simulink model "base_evaluation_1008_24b"  (R2016b)
settings: Solver=FixedStepAuto  StartTime=0.0  StopTime=10.0  RelTol=1e-3
settings Model: Creator=Cheng  LastModifiedBy=kensh
settings DataIOCC: ReturnWorkspaceOutputs=on
settings OptimizationCC: DefaultParameterBehavior=Inlined
settings DebuggingCC: ParameterTunabilityLossMsg=error  UnconnectedInputMsg=none  UnconnectedOutputMsg=none  UnconnectedLineMsg=none
settings ModelReferenceCC: EnableRefExpFcnMdlSchedulingChecks=off
settings SFSimCC: SimUseLocalCustomCode=on
settings RTWCC: SystemTargetFile=ert.tlc  TemplateMakefile=ert_default_tmf  Description=Embedded Coder  GenerateReport=on  RTWUseLocalCustomCode=on  IncludeHyperlinkInReport=on  LaunchReport=on  GenerateTraceInfo=on  GenerateTraceReport=on  GenerateTraceReportSl=on  GenerateTraceReportSf=on  GenerateTraceReportEml=on
settings CodeAppCC: ForceParamTrailComments=on  IgnoreCustomStorageClasses=off  OperatorAnnotations=on  SimulinkDataObjDesc=on  SFDataObjDesc=on  MATLABFcnDesc=on  InsertBlockDesc=on  MATLABSourceComments=on
settings ERTTargetCC: TargetLangStandard=C99 (ISO)  GenerateSampleERTMain=on  InlinedParameterPlacement=NonHierarchical  ERTCustomFileTemplate=example_file_process.tlc

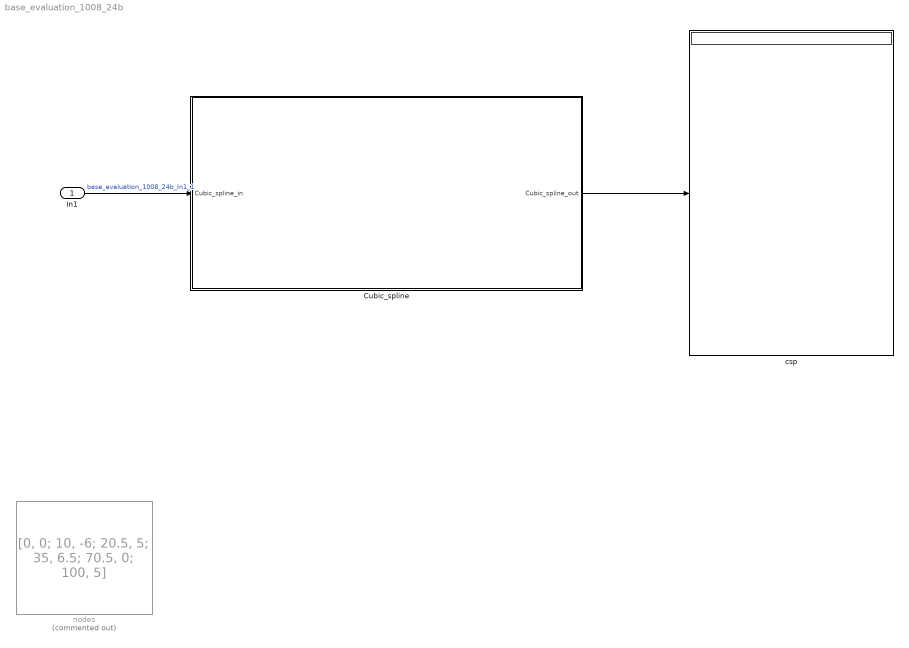
== system base_evaluation_1008_24b ==
  In1 : Inport
  Cubic_spline : Subsystem
  csp : Display
  nodes : Constant  Commented=on  Value=[0, 0; 10, -6; 20.5, 5; 35, 6.5; 70.5, 0; 100, 5]
  wires:
  Cubic_spline/1(Cubic_spline_out) -> csp/1
  In1/1 -> Cubic_spline/1(Cubic_spline_in)  "base_evaluation_1008_24b_In1_1"

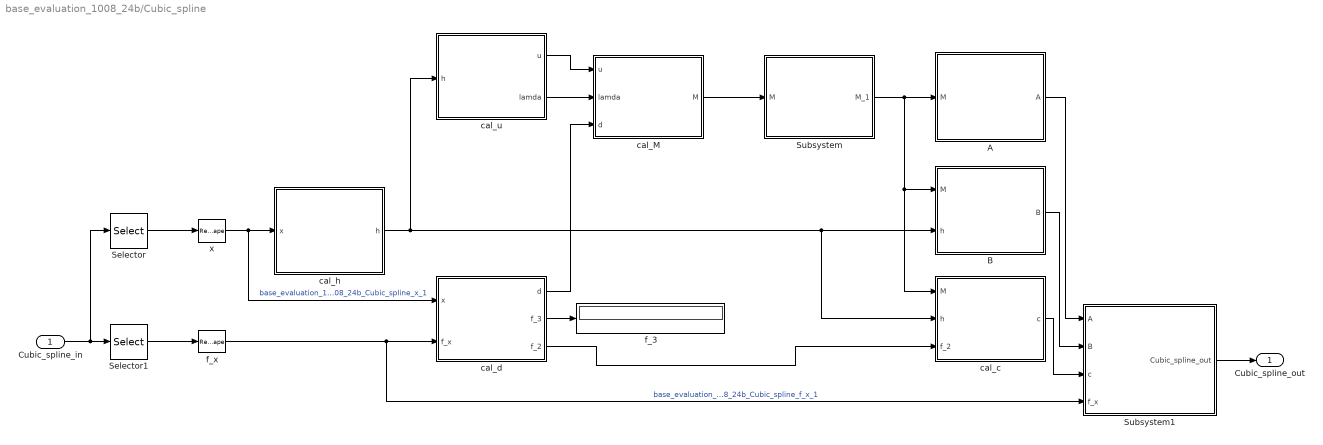
== system base_evaluation_1008_24b/Cubic_spline ==
  Cubic_spline_in : Inport
  A : Subsystem
  B : Subsystem
  Selector : Selector  NumberOfDimensions=2  InputPortWidth=3  IndexOptions=Select all,Index vector (dialog)  Indices=1,1  OutputSizes=1,1
  Selector1 : Selector  NumberOfDimensions=2  InputPortWidth=3  IndexOptions=Select all,Index vector (dialog)  Indices=1,2  OutputSizes=1,1
  Subsystem : Subsystem
  Subsystem1 : Subsystem
  cal_M : Subsystem
  cal_c : Subsystem
  cal_d : Subsystem
  cal_h : Subsystem
  cal_u : Subsystem
  f_3 : Display
  f_x : Reshape  OutputDimensionality=Row vector (2-D)
  x : Reshape  OutputDimensionality=Row vector (2-D)
  Cubic_spline_out : Outport
  wires:
  Cubic_spline_in/1 -> Selector1/1, Selector/1
  f_x/1 -> Subsystem1/4(f_x), cal_d/2(f_x)  "base_evaluation_1008_24b_Cubic_spline_f_x_1"
  Selector1/1 -> f_x/1
  Selector/1 -> x/1
  x/1 -> cal_d/1(x), cal_h/1(x)  "base_evaluation_1008_24b_Cubic_spline_x_1"
  cal_M/1(M) -> Subsystem/1(M)
  cal_h/1(h) -> cal_c/2(h), B/2(h), cal_u/1(h)
  cal_u/1(u) -> cal_M/1(u)
  cal_c/1(c) -> Subsystem1/3(c)
  cal_u/2(lamda) -> cal_M/2(lamda)
  cal_d/1(d) -> cal_M/3(d)
  cal_d/2(f_3) -> f_3/1
  cal_d/3(f_2) -> cal_c/3(f_2)
  Subsystem/1(M_1) -> B/1(M), cal_c/1(M), A/1(M)
  A/1(A) -> Subsystem1/1(A)
  B/1(B) -> Subsystem1/2(B)
  Subsystem1/1(Cubic_spline_out) -> Cubic_spline_out/1

== system base_evaluation_1008_24b/Cubic_spline/A ==
  M : Inport
  Gain{,1..4} (5 alike) : Gain  Gain=0.5
  M1 : Selector  InputPortWidth=6  IndexOptions=Index vector (dialog)  Indices=[1]  OutputSizes=1
  M2 : Selector  InputPortWidth=6  IndexOptions=Index vector (dialog)  Indices=[2]  OutputSizes=1
  M3 : Selector  InputPortWidth=6  IndexOptions=Index vector (dialog)  Indices=[3]  OutputSizes=1
  M4 : Selector  InputPortWidth=6  IndexOptions=Index vector (dialog)  Indices=[4]  OutputSizes=1
  M5 : Selector  InputPortWidth=6  IndexOptions=Index vector (dialog)  Indices=[5]  OutputSizes=1
  Mux : Mux  Inputs=5
  Reshape : Reshape  OutputDimensionality=Row vector (2-D)
  A : Outport
  wires:
  M3/1 -> Gain2/1
  M4/1 -> Gain3/1
  M/1 -> M5/1, M4/1, M3/1, M2/1, M1/1
  M2/1 -> Gain1/1
  M1/1 -> Gain/1
  M5/1 -> Gain4/1
  Gain/1 -> Mux/1  "base_evaluation_1008_24b_Cubic_spline_A_Gain_1"
  Gain1/1 -> Mux/2  "base_evaluation_1008_24b_Cubic_spline_A_Gain1_1"
  Gain2/1 -> Mux/3  "base_evaluation_1008_24b_Cubic_spline_A_Gain2_1"
  Gain3/1 -> Mux/4  "base_evaluation_1008_24b_Cubic_spline_A_Gain3_1"
  Gain4/1 -> Mux/5  "base_evaluation_1008_24b_Cubic_spline_A_Gain4_1"
  Mux/1 -> Reshape/1
  Reshape/1 -> A/1  "base_evaluation_1008_24b_Cubic_spline_A_Reshape_1"

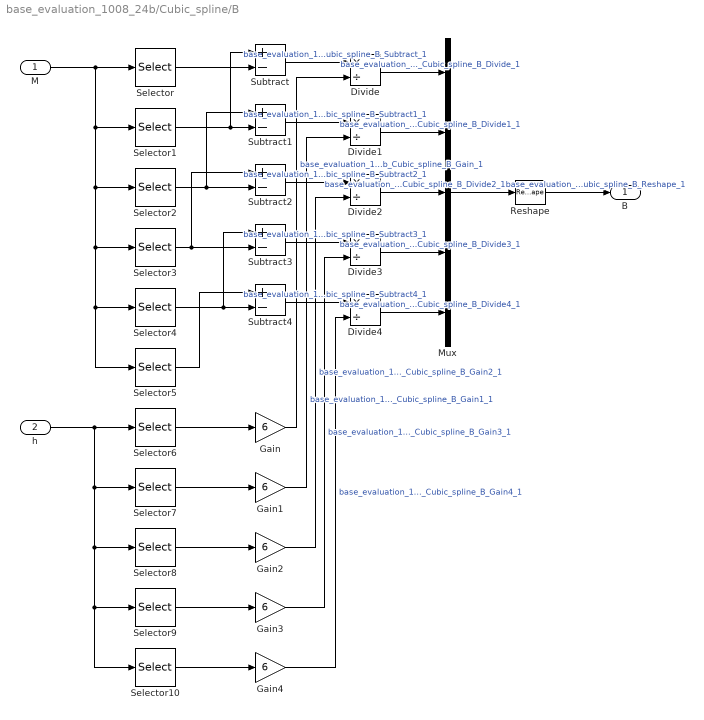
== system base_evaluation_1008_24b/Cubic_spline/B ==
  M : Inport
  h : Inport  Port=2
  Divide{,1..4} (5 alike) : Product  Inputs=*/
  Gain{,1..4} (5 alike) : Gain  Gain=6
  Mux : Mux  Inputs=5
  Reshape : Reshape  OutputDimensionality=Row vector (2-D)
  Selector : Selector  InputPortWidth=6  IndexOptions=Index vector (dialog)  Indices=[1]  OutputSizes=1
  Selector1 : Selector  InputPortWidth=6  IndexOptions=Index vector (dialog)  Indices=[2]  OutputSizes=1
  Selector10 : Selector  InputPortWidth=5  IndexOptions=Index vector (dialog)  Indices=[5]  OutputSizes=1
  Selector2 : Selector  InputPortWidth=6  IndexOptions=Index vector (dialog)  Indices=[3]  OutputSizes=1
  Selector3 : Selector  InputPortWidth=6  IndexOptions=Index vector (dialog)  Indices=[4]  OutputSizes=1
  Selector4 : Selector  InputPortWidth=6  IndexOptions=Index vector (dialog)  Indices=[5]  OutputSizes=1
  Selector5 : Selector  InputPortWidth=6  IndexOptions=Index vector (dialog)  Indices=[6]  OutputSizes=1
  Selector6 : Selector  InputPortWidth=5  IndexOptions=Index vector (dialog)  Indices=[1]  OutputSizes=1
  Selector7 : Selector  InputPortWidth=5  IndexOptions=Index vector (dialog)  Indices=[2]  OutputSizes=1
  Selector8 : Selector  InputPortWidth=5  IndexOptions=Index vector (dialog)  Indices=[3]  OutputSizes=1
  Selector9 : Selector  InputPortWidth=5  IndexOptions=Index vector (dialog)  Indices=[4]  OutputSizes=1
  Subtract{,1..4} (5 alike) : Sum  Inputs=+-
  B : Outport
  wires:
  h/1 -> Selector10/1, Selector9/1, Selector8/1, Selector7/1, Selector6/1
  M/1 -> Selector5/1, Selector4/1, Selector3/1, Selector2/1, Selector1/1, Selector/1
  Selector1/1 -> Subtract1/2, Subtract/1
  Selector/1 -> Subtract/2
  Selector2/1 -> Subtract2/2, Subtract1/1
  Selector3/1 -> Subtract3/2, Subtract2/1
  Selector6/1 -> Gain/1
  Selector7/1 -> Gain1/1
  Selector8/1 -> Gain2/1
  Subtract/1 -> Divide/1  "base_evaluation_1008_24b_Cubic_spline_B_Subtract_1"
  Gain/1 -> Divide/2  "base_evaluation_1008_24b_Cubic_spline_B_Gain_1"
  Subtract1/1 -> Divide1/1  "base_evaluation_1008_24b_Cubic_spline_B_Subtract1_1"
  Gain1/1 -> Divide1/2  "base_evaluation_1008_24b_Cubic_spline_B_Gain1_1"
  Subtract2/1 -> Divide2/1  "base_evaluation_1008_24b_Cubic_spline_B_Subtract2_1"
  Gain2/1 -> Divide2/2  "base_evaluation_1008_24b_Cubic_spline_B_Gain2_1"
  Divide/1 -> Mux/1  "base_evaluation_1008_24b_Cubic_spline_B_Divide_1"
  Divide1/1 -> Mux/2  "base_evaluation_1008_24b_Cubic_spline_B_Divide1_1"
  Divide2/1 -> Mux/3  "base_evaluation_1008_24b_Cubic_spline_B_Divide2_1"
  Mux/1 -> Reshape/1
  Reshape/1 -> B/1  "base_evaluation_1008_24b_Cubic_spline_B_Reshape_1"
  Selector4/1 -> Subtract4/2, Subtract3/1
  Selector5/1 -> Subtract4/1
  Selector9/1 -> Gain3/1
  Selector10/1 -> Gain4/1
  Divide3/1 -> Mux/4  "base_evaluation_1008_24b_Cubic_spline_B_Divide3_1"
  Divide4/1 -> Mux/5  "base_evaluation_1008_24b_Cubic_spline_B_Divide4_1"
  Subtract3/1 -> Divide3/1  "base_evaluation_1008_24b_Cubic_spline_B_Subtract3_1"
  Subtract4/1 -> Divide4/1  "base_evaluation_1008_24b_Cubic_spline_B_Subtract4_1"
  Gain3/1 -> Divide3/2  "base_evaluation_1008_24b_Cubic_spline_B_Gain3_1"
  Gain4/1 -> Divide4/2  "base_evaluation_1008_24b_Cubic_spline_B_Gain4_1"

== system base_evaluation_1008_24b/Cubic_spline/Subsystem ==
  M : Inport
  Constant : Constant  Value=0
  Constant1 : Constant  Value=0
  M1 : Selector  InputPortWidth=4  IndexOptions=Index vector (dialog)  Indices=[1]  OutputSizes=1
  M2 : Selector  InputPortWidth=4  IndexOptions=Index vector (dialog)  Indices=[2]  OutputSizes=1
  M3 : Selector  InputPortWidth=4  IndexOptions=Index vector (dialog)  Indices=[3]  OutputSizes=1
  M4 : Selector  InputPortWidth=4  IndexOptions=Index vector (dialog)  Indices=[4]  OutputSizes=1
  Mux : Mux  Inputs=6
  Reshape : Reshape  OutputDimensionality=Column vector (2-D)
  M_1 : Outport
  wires:
  Mux/1 -> Reshape/1
  Constant/1 -> Mux/1  "base_evaluation_1008_24b_Cubic_spline_Subsystem_Constant_1"
  M1/1 -> Mux/2
  Constant1/1 -> Mux/6  "base_evaluation_1008_24b_Cubic_spline_Subsystem_Constant1_1"
  M2/1 -> Mux/3
  Reshape/1 -> M_1/1  "base_evaluation_1008_24b_Cubic_spline_Subsystem_Reshape_1"
  M3/1 -> Mux/4
  M4/1 -> Mux/5
  M/1 -> M4/1, M3/1, M2/1, M1/1

== system base_evaluation_1008_24b/Cubic_spline/Subsystem1 ==
  A : Inport
  B : Inport  Port=2
  c : Inport  Port=3
  f_x : Inport  Port=4
  MatrixConcatenate : Concatenate  NumInputs=5  Mode=Multidimensional array
  Subsystem : Subsystem
  Subsystem1 : Subsystem
  Subsystem2 : Subsystem
  Subsystem3 : Subsystem
  Subsystem4 : Subsystem
  Cubic_spline_out : Outport
  wires:
  A/1 -> Subsystem1/1(A), Subsystem2/1(A), Subsystem4/1(A), Subsystem3/1(A), Subsystem/1(A)
  B/1 -> Subsystem/2(B), Subsystem1/2(B), Subsystem2/2(B), Subsystem4/2(B), Subsystem3/2(B)
  c/1 -> Subsystem/3(c), Subsystem1/3(c), Subsystem2/3(c), Subsystem4/3(c), Subsystem3/3(c)
  f_x/1 -> Subsystem/4(f_x), Subsystem1/4(f_x), Subsystem2/4(f_x), Subsystem4/4(f_x), Subsystem3/4(f_x)
  Subsystem/1(1) -> MatrixConcatenate/1
  Subsystem1/1(2) -> MatrixConcatenate/2
  Subsystem2/1(3) -> MatrixConcatenate/3
  Subsystem3/1(4) -> MatrixConcatenate/4
  Subsystem4/1(5) -> MatrixConcatenate/5
  MatrixConcatenate/1 -> Cubic_spline_out/1  "base_evaluation_1008_24b_Cubic_spline_Subsystem1_MatrixConcatenate_1"

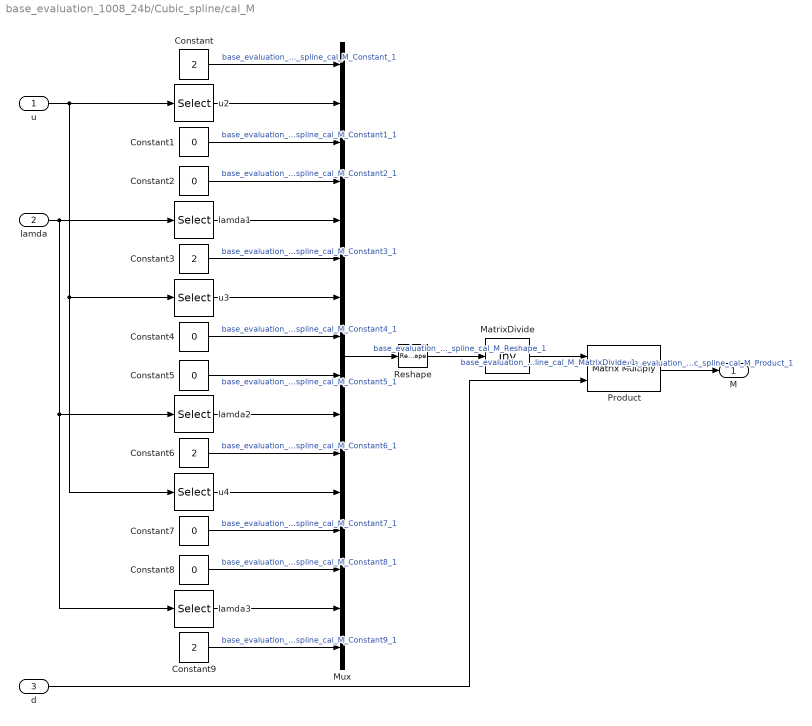
== system base_evaluation_1008_24b/Cubic_spline/cal_M ==
  u : Inport
  lamda : Inport  Port=2
  d : Inport  Port=3
  Constant{,3,6,9} (4 alike) : Constant  Value=2
  Constant{1..2,4..5,7..8} (6 alike) : Constant  Value=0
  MatrixDivide : Product  Inputs=/  Multiplication=Matrix(*)
  Mux : Mux  Inputs=16
  Product : Product  Multiplication=Matrix(*)
  Reshape : Reshape  OutputDimensionality=Customize  OutputDimensions=[4,4]
  lamda1 : Selector  InputPortWidth=4  IndexOptions=Index vector (dialog)  Indices=[1]  OutputSizes=1
  lamda2 : Selector  InputPortWidth=4  IndexOptions=Index vector (dialog)  Indices=[2]  OutputSizes=1
  lamda3 : Selector  InputPortWidth=4  IndexOptions=Index vector (dialog)  Indices=[3]  OutputSizes=1
  u2 : Selector  InputPortWidth=4  IndexOptions=Index vector (dialog)  Indices=[2]  OutputSizes=1
  u3 : Selector  InputPortWidth=4  IndexOptions=Index vector (dialog)  Indices=[3]  OutputSizes=1
  u4 : Selector  InputPortWidth=4  IndexOptions=Index vector (dialog)  Indices=[4]  OutputSizes=1
  M : Outport
  wires:
  u/1 -> u2/1, u4/1, u3/1
  Mux/1 -> Reshape/1
  Constant/1 -> Mux/1  "base_evaluation_1008_24b_Cubic_spline_cal_M_Constant_1"
  Product/1 -> M/1  "base_evaluation_1008_24b_Cubic_spline_cal_M_Product_1"
  Constant1/1 -> Mux/3  "base_evaluation_1008_24b_Cubic_spline_cal_M_Constant1_1"
  Constant2/1 -> Mux/4  "base_evaluation_1008_24b_Cubic_spline_cal_M_Constant2_1"
  u2/1 -> Mux/2
  lamda1/1 -> Mux/5
  Constant3/1 -> Mux/6  "base_evaluation_1008_24b_Cubic_spline_cal_M_Constant3_1"
  u3/1 -> Mux/7
  Constant4/1 -> Mux/8  "base_evaluation_1008_24b_Cubic_spline_cal_M_Constant4_1"
  Constant5/1 -> Mux/9  "base_evaluation_1008_24b_Cubic_spline_cal_M_Constant5_1"
  lamda/1 -> lamda3/1, lamda2/1, lamda1/1
  lamda2/1 -> Mux/10
  Constant6/1 -> Mux/11  "base_evaluation_1008_24b_Cubic_spline_cal_M_Constant6_1"
  u4/1 -> Mux/12
  Constant7/1 -> Mux/13  "base_evaluation_1008_24b_Cubic_spline_cal_M_Constant7_1"
  Constant8/1 -> Mux/14  "base_evaluation_1008_24b_Cubic_spline_cal_M_Constant8_1"
  lamda3/1 -> Mux/15
  Constant9/1 -> Mux/16  "base_evaluation_1008_24b_Cubic_spline_cal_M_Constant9_1"
  Reshape/1 -> MatrixDivide/1  "base_evaluation_1008_24b_Cubic_spline_cal_M_Reshape_1"
  d/1 -> Product/2
  MatrixDivide/1 -> Product/1  "base_evaluation_1008_24b_Cubic_spline_cal_M_MatrixDivide_1"

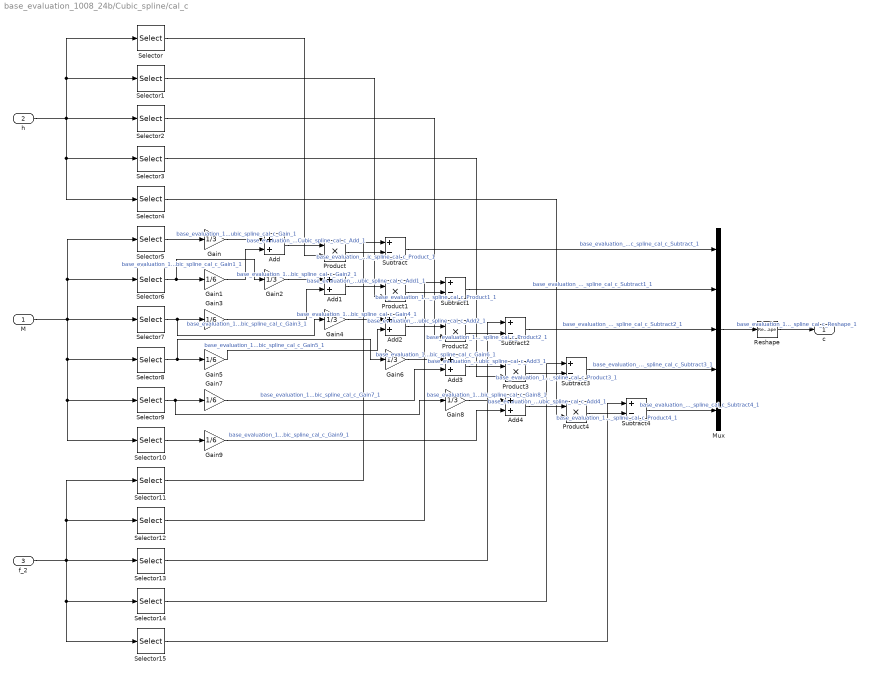
== system base_evaluation_1008_24b/Cubic_spline/cal_c ==
  M : Inport
  h : Inport  Port=2
  f_2 : Inport  Port=3
  Add{,1..4} (5 alike) : Sum
  Gain{,2,4,6,8} (5 alike) : Gain  Gain=1/3
  Gain{1,3,5,7,9} (5 alike) : Gain  Gain=1/6
  Mux : Mux  Inputs=5
  Product{,1..4} (5 alike) : Product
  Reshape : Reshape  OutputDimensionality=Row vector (2-D)
  Selector : Selector  InputPortWidth=5  IndexOptions=Index vector (dialog)  Indices=[1]  OutputSizes=1
  Selector1 : Selector  InputPortWidth=5  IndexOptions=Index vector (dialog)  Indices=[2]  OutputSizes=1
  Selector10 : Selector  InputPortWidth=6  IndexOptions=Index vector (dialog)  Indices=[6]  OutputSizes=1
  Selector11 : Selector  InputPortWidth=5  IndexOptions=Index vector (dialog)  Indices=[1]  OutputSizes=1
  Selector12 : Selector  InputPortWidth=5  IndexOptions=Index vector (dialog)  Indices=[2]  OutputSizes=1
  Selector13 : Selector  InputPortWidth=5  IndexOptions=Index vector (dialog)  Indices=[3]  OutputSizes=1
  Selector14 : Selector  InputPortWidth=5  IndexOptions=Index vector (dialog)  Indices=[4]  OutputSizes=1
  Selector15 : Selector  InputPortWidth=5  IndexOptions=Index vector (dialog)  Indices=[5]  OutputSizes=1
  Selector2 : Selector  InputPortWidth=5  IndexOptions=Index vector (dialog)  Indices=[3]  OutputSizes=1
  Selector3 : Selector  InputPortWidth=5  IndexOptions=Index vector (dialog)  Indices=[4]  OutputSizes=1
  Selector4 : Selector  InputPortWidth=5  IndexOptions=Index vector (dialog)  Indices=[5]  OutputSizes=1
  Selector5 : Selector  InputPortWidth=6  IndexOptions=Index vector (dialog)  Indices=[1]  OutputSizes=1
  Selector6 : Selector  InputPortWidth=6  IndexOptions=Index vector (dialog)  Indices=[2]  OutputSizes=1
  Selector7 : Selector  InputPortWidth=6  IndexOptions=Index vector (dialog)  Indices=[3]  OutputSizes=1
  Selector8 : Selector  InputPortWidth=6  IndexOptions=Index vector (dialog)  Indices=[4]  OutputSizes=1
  Selector9 : Selector  InputPortWidth=6  IndexOptions=Index vector (dialog)  Indices=[5]  OutputSizes=1
  Subtract{,1..4} (5 alike) : Sum  Inputs=+-
  c : Outport
  wires:
  Selector2/1 -> Product2/2
  Selector6/1 -> Gain2/1, Gain1/1
  Gain3/1 -> Add1/2  "base_evaluation_1008_24b_Cubic_spline_cal_c_Gain3_1"
  Gain/1 -> Add/1  "base_evaluation_1008_24b_Cubic_spline_cal_c_Gain_1"
  Selector7/1 -> Gain3/1, Gain4/1
  f_2/1 -> Selector11/1, Selector12/1, Selector15/1, Selector14/1, Selector13/1
  Add1/1 -> Product1/1  "base_evaluation_1008_24b_Cubic_spline_cal_c_Add1_1"
  Selector1/1 -> Product1/2
  M/1 -> Selector8/1, Selector9/1, Selector10/1, Selector7/1, Selector6/1, Selector5/1
  Subtract1/1 -> Mux/2  "base_evaluation_1008_24b_Cubic_spline_cal_c_Subtract1_1"
  Reshape/1 -> c/1  "base_evaluation_1008_24b_Cubic_spline_cal_c_Reshape_1"
  Gain1/1 -> Add/2  "base_evaluation_1008_24b_Cubic_spline_cal_c_Gain1_1"
  Add2/1 -> Product2/1  "base_evaluation_1008_24b_Cubic_spline_cal_c_Add2_1"
  Selector/1 -> Product/2
  Gain2/1 -> Add1/1  "base_evaluation_1008_24b_Cubic_spline_cal_c_Gain2_1"
  Selector5/1 -> Gain/1
  Subtract/1 -> Mux/1  "base_evaluation_1008_24b_Cubic_spline_cal_c_Subtract_1"
  Subtract2/1 -> Mux/3  "base_evaluation_1008_24b_Cubic_spline_cal_c_Subtract2_1"
  Selector13/1 -> Subtract2/1
  Gain4/1 -> Add2/1  "base_evaluation_1008_24b_Cubic_spline_cal_c_Gain4_1"
  Add/1 -> Product/1  "base_evaluation_1008_24b_Cubic_spline_cal_c_Add_1"
  Selector12/1 -> Subtract1/1
  h/1 -> Selector4/1, Selector3/1, Selector/1, Selector1/1, Selector2/1
  Selector11/1 -> Subtract/1
  Product2/1 -> Subtract2/2  "base_evaluation_1008_24b_Cubic_spline_cal_c_Product2_1"
  Product1/1 -> Subtract1/2  "base_evaluation_1008_24b_Cubic_spline_cal_c_Product1_1"
  Selector8/1 -> Gain6/1, Gain5/1
  Mux/1 -> Reshape/1
  Gain5/1 -> Add2/2  "base_evaluation_1008_24b_Cubic_spline_cal_c_Gain5_1"
  Product/1 -> Subtract/2  "base_evaluation_1008_24b_Cubic_spline_cal_c_Product_1"
  Selector9/1 -> Gain8/1, Gain7/1
  Gain6/1 -> Add3/1  "base_evaluation_1008_24b_Cubic_spline_cal_c_Gain6_1"
  Gain7/1 -> Add3/2  "base_evaluation_1008_24b_Cubic_spline_cal_c_Gain7_1"
  Add3/1 -> Product3/1  "base_evaluation_1008_24b_Cubic_spline_cal_c_Add3_1"
  Selector3/1 -> Product3/2
  Product3/1 -> Subtract3/2  "base_evaluation_1008_24b_Cubic_spline_cal_c_Product3_1"
  Selector14/1 -> Subtract3/1
  Selector10/1 -> Gain9/1
  Gain9/1 -> Add4/2  "base_evaluation_1008_24b_Cubic_spline_cal_c_Gain9_1"
  Gain8/1 -> Add4/1  "base_evaluation_1008_24b_Cubic_spline_cal_c_Gain8_1"
  Add4/1 -> Product4/1  "base_evaluation_1008_24b_Cubic_spline_cal_c_Add4_1"
  Selector4/1 -> Product4/2
  Product4/1 -> Subtract4/2  "base_evaluation_1008_24b_Cubic_spline_cal_c_Product4_1"
  Subtract3/1 -> Mux/4  "base_evaluation_1008_24b_Cubic_spline_cal_c_Subtract3_1"
  Selector15/1 -> Subtract4/1
  Subtract4/1 -> Mux/5  "base_evaluation_1008_24b_Cubic_spline_cal_c_Subtract4_1"

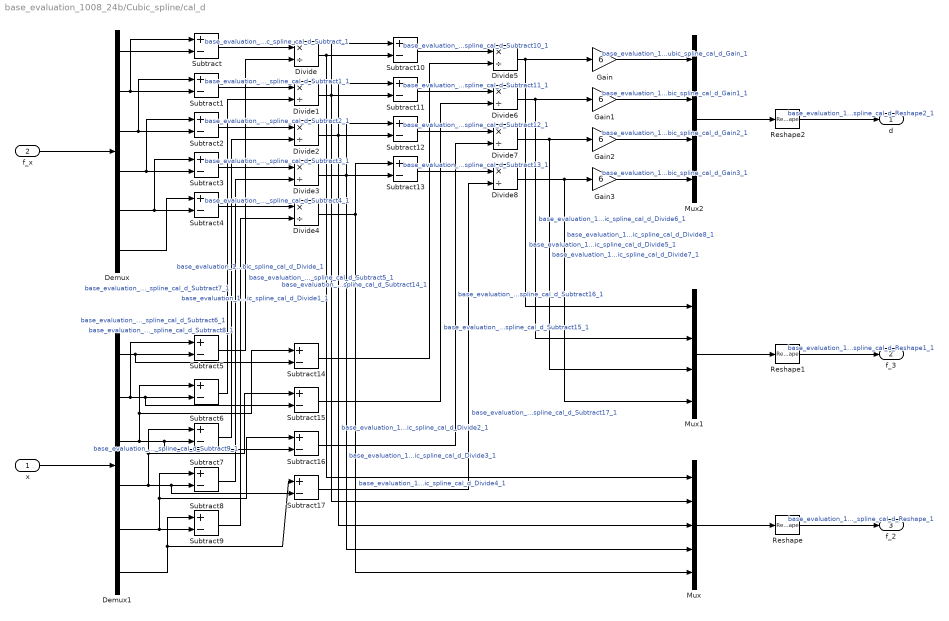
== system base_evaluation_1008_24b/Cubic_spline/cal_d ==
  x : Inport
  f_x : Inport  Port=2
  Demux : Demux  Outputs=6
  Demux1 : Demux  Outputs=6
  Divide{,1..8} (9 alike) : Product  Inputs=*/
  Gain{,1..3} (4 alike) : Gain  Gain=6
  Mux : Mux  Inputs=5
  Mux1 : Mux
  Mux2 : Mux
  Reshape : Reshape  OutputDimensionality=Row vector (2-D)
  Reshape1 : Reshape  OutputDimensionality=Row vector (2-D)
  Reshape2 : Reshape  OutputDimensionality=Column vector (2-D)
  Subtract{,1..17} (18 alike) : Sum  Inputs=+-
  d : Outport
  f_3 : Outport  Port=2
  f_2 : Outport  Port=3
  wires:
  f_x/1 -> Demux/1
  Demux1/2 -> Subtract6/2, Subtract15/2, Subtract5/1
  Demux/2 -> Subtract1/2, Subtract/1
  Mux/1 -> Reshape/1
  Subtract11/1 -> Divide6/1  "base_evaluation_1008_24b_Cubic_spline_cal_d_Subtract11_1"
  Subtract1/1 -> Divide1/1  "base_evaluation_1008_24b_Cubic_spline_cal_d_Subtract1_1"
  Demux/4 -> Subtract3/2, Subtract2/1
  Demux1/1 -> Subtract14/2, Subtract5/2
  Mux1/1 -> Reshape1/1
  Demux/3 -> Subtract2/2, Subtract1/1
  Divide2/1 -> Mux/3, Subtract12/2, Subtract11/1  "base_evaluation_1008_24b_Cubic_spline_cal_d_Divide2_1"
  Reshape1/1 -> f_3/1  "base_evaluation_1008_24b_Cubic_spline_cal_d_Reshape1_1"
  Divide1/1 -> Mux/2, Subtract11/2, Subtract10/1  "base_evaluation_1008_24b_Cubic_spline_cal_d_Divide1_1"
  Divide/1 -> Subtract10/2, Mux/1  "base_evaluation_1008_24b_Cubic_spline_cal_d_Divide_1"
  Divide6/1 -> Gain1/1, Mux1/2  "base_evaluation_1008_24b_Cubic_spline_cal_d_Divide6_1"
  Divide5/1 -> Gain/1, Mux1/1  "base_evaluation_1008_24b_Cubic_spline_cal_d_Divide5_1"
  Demux1/4 -> Subtract17/2, Subtract8/2, Subtract7/1, Subtract15/1
  Subtract6/1 -> Divide1/2  "base_evaluation_1008_24b_Cubic_spline_cal_d_Subtract6_1"
  Subtract10/1 -> Divide5/1  "base_evaluation_1008_24b_Cubic_spline_cal_d_Subtract10_1"
  Subtract2/1 -> Divide2/1  "base_evaluation_1008_24b_Cubic_spline_cal_d_Subtract2_1"
  Demux/1 -> Subtract/2
  Reshape2/1 -> d/1  "base_evaluation_1008_24b_Cubic_spline_cal_d_Reshape2_1"
  Subtract/1 -> Divide/1  "base_evaluation_1008_24b_Cubic_spline_cal_d_Subtract_1"
  Subtract15/1 -> Divide6/2  "base_evaluation_1008_24b_Cubic_spline_cal_d_Subtract15_1"
  Subtract14/1 -> Divide5/2  "base_evaluation_1008_24b_Cubic_spline_cal_d_Subtract14_1"
  x/1 -> Demux1/1
  Subtract5/1 -> Divide/2  "base_evaluation_1008_24b_Cubic_spline_cal_d_Subtract5_1"
  Reshape/1 -> f_2/1  "base_evaluation_1008_24b_Cubic_spline_cal_d_Reshape_1"
  Demux1/3 -> Subtract16/2, Subtract7/2, Subtract14/1, Subtract6/1
  Mux2/1 -> Reshape2/1
  Subtract7/1 -> Divide2/2  "base_evaluation_1008_24b_Cubic_spline_cal_d_Subtract7_1"
  Demux/5 -> Subtract3/1, Subtract4/2
  Demux/6 -> Subtract4/1
  Demux1/5 -> Subtract9/2, Subtract8/1, Subtract16/1
  Demux1/6 -> Subtract9/1, Subtract17/1
  Subtract3/1 -> Divide3/1  "base_evaluation_1008_24b_Cubic_spline_cal_d_Subtract3_1"
  Subtract8/1 -> Divide3/2  "base_evaluation_1008_24b_Cubic_spline_cal_d_Subtract8_1"
  Subtract4/1 -> Divide4/1  "base_evaluation_1008_24b_Cubic_spline_cal_d_Subtract4_1"
  Subtract9/1 -> Divide4/2  "base_evaluation_1008_24b_Cubic_spline_cal_d_Subtract9_1"
  Divide4/1 -> Subtract13/1, Mux/5  "base_evaluation_1008_24b_Cubic_spline_cal_d_Divide4_1"
  Subtract12/1 -> Divide7/1  "base_evaluation_1008_24b_Cubic_spline_cal_d_Subtract12_1"
  Subtract13/1 -> Divide8/1  "base_evaluation_1008_24b_Cubic_spline_cal_d_Subtract13_1"
  Subtract16/1 -> Divide7/2  "base_evaluation_1008_24b_Cubic_spline_cal_d_Subtract16_1"
  Subtract17/1 -> Divide8/2  "base_evaluation_1008_24b_Cubic_spline_cal_d_Subtract17_1"
  Divide7/1 -> Gain2/1, Mux1/3  "base_evaluation_1008_24b_Cubic_spline_cal_d_Divide7_1"
  Divide8/1 -> Gain3/1, Mux1/4  "base_evaluation_1008_24b_Cubic_spline_cal_d_Divide8_1"
  Divide3/1 -> Mux/4, Subtract13/2, Subtract12/1  "base_evaluation_1008_24b_Cubic_spline_cal_d_Divide3_1"
  Gain/1 -> Mux2/1  "base_evaluation_1008_24b_Cubic_spline_cal_d_Gain_1"
  Gain1/1 -> Mux2/2  "base_evaluation_1008_24b_Cubic_spline_cal_d_Gain1_1"
  Gain2/1 -> Mux2/3  "base_evaluation_1008_24b_Cubic_spline_cal_d_Gain2_1"
  Gain3/1 -> Mux2/4  "base_evaluation_1008_24b_Cubic_spline_cal_d_Gain3_1"

== system base_evaluation_1008_24b/Cubic_spline/cal_h ==
  x : Inport
  Demux : Demux  Outputs=6
  Mux : Mux  Inputs=5
  Reshape : Reshape  OutputDimensionality=Row vector (2-D)
  Subtract{,1..4} (5 alike) : Sum  Inputs=+-
  h : Outport
  wires:
  Mux/1 -> Reshape/1
  Subtract1/1 -> Mux/2  "base_evaluation_1008_24b_Cubic_spline_cal_h_Subtract1_1"
  Demux/1 -> Subtract/2
  x/1 -> Demux/1
  Demux/3 -> Subtract1/1, Subtract2/2
  Demux/4 -> Subtract2/1, Subtract3/2
  Reshape/1 -> h/1  "base_evaluation_1008_24b_Cubic_spline_cal_h_Reshape_1"
  Demux/2 -> Subtract1/2, Subtract/1
  Subtract2/1 -> Mux/3  "base_evaluation_1008_24b_Cubic_spline_cal_h_Subtract2_1"
  Demux/5 -> Subtract3/1, Subtract4/2
  Demux/6 -> Subtract4/1
  Subtract3/1 -> Mux/4  "base_evaluation_1008_24b_Cubic_spline_cal_h_Subtract3_1"
  Subtract4/1 -> Mux/5  "base_evaluation_1008_24b_Cubic_spline_cal_h_Subtract4_1"
  Subtract/1 -> Mux/1  "base_evaluation_1008_24b_Cubic_spline_cal_h_Subtract_1"

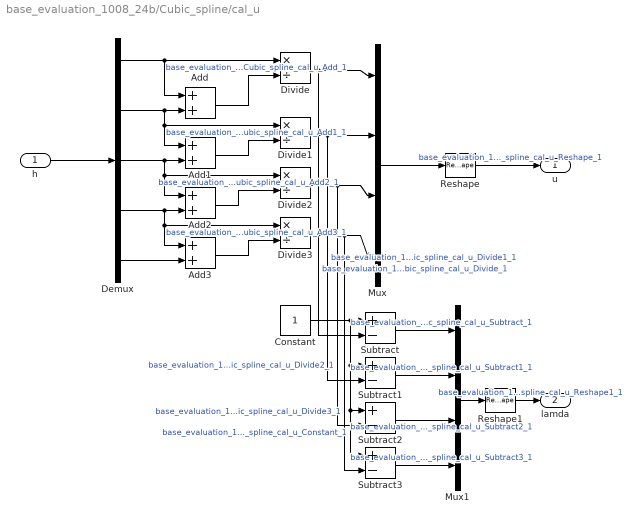
== system base_evaluation_1008_24b/Cubic_spline/cal_u ==
  h : Inport
  Add{,1..3} (4 alike) : Sum
  Constant : Constant
  Demux : Demux  Outputs=5
  Divide{,1..3} (4 alike) : Product  Inputs=*/
  Mux : Mux
  Mux1 : Mux
  Reshape : Reshape  OutputDimensionality=Row vector (2-D)
  Reshape1 : Reshape  OutputDimensionality=Row vector (2-D)
  Subtract{,1..3} (4 alike) : Sum  Inputs=+-
  u : Outport
  lamda : Outport  Port=2
  wires:
  Reshape1/1 -> lamda/1  "base_evaluation_1008_24b_Cubic_spline_cal_u_Reshape1_1"
  Demux/3 -> Divide2/1, Add2/1, Add1/2
  Mux/1 -> Reshape/1
  Add1/1 -> Divide1/2  "base_evaluation_1008_24b_Cubic_spline_cal_u_Add1_1"
  Demux/2 -> Add1/1, Divide1/1, Add/2
  h/1 -> Demux/1
  Constant/1 -> Subtract3/1, Subtract2/1, Subtract1/1, Subtract/1  "base_evaluation_1008_24b_Cubic_spline_cal_u_Constant_1"
  Reshape/1 -> u/1  "base_evaluation_1008_24b_Cubic_spline_cal_u_Reshape_1"
  Demux/1 -> Divide/1, Add/1
  Subtract/1 -> Mux1/1  "base_evaluation_1008_24b_Cubic_spline_cal_u_Subtract_1"
  Subtract1/1 -> Mux1/2  "base_evaluation_1008_24b_Cubic_spline_cal_u_Subtract1_1"
  Mux1/1 -> Reshape1/1
  Demux/4 -> Divide3/1, Add3/1, Add2/2
  Demux/5 -> Add3/2
  Add2/1 -> Divide2/2  "base_evaluation_1008_24b_Cubic_spline_cal_u_Add2_1"
  Add3/1 -> Divide3/2  "base_evaluation_1008_24b_Cubic_spline_cal_u_Add3_1"
  Subtract2/1 -> Mux1/3  "base_evaluation_1008_24b_Cubic_spline_cal_u_Subtract2_1"
  Subtract3/1 -> Mux1/4  "base_evaluation_1008_24b_Cubic_spline_cal_u_Subtract3_1"
  Add/1 -> Divide/2  "base_evaluation_1008_24b_Cubic_spline_cal_u_Add_1"
  Divide/1 -> Subtract/2, Mux/1  "base_evaluation_1008_24b_Cubic_spline_cal_u_Divide_1"
  Divide1/1 -> Subtract1/2, Mux/2  "base_evaluation_1008_24b_Cubic_spline_cal_u_Divide1_1"
  Divide2/1 -> Subtract2/2, Mux/3  "base_evaluation_1008_24b_Cubic_spline_cal_u_Divide2_1"
  Divide3/1 -> Subtract3/2, Mux/4  "base_evaluation_1008_24b_Cubic_spline_cal_u_Divide3_1"

== system base_evaluation_1008_24b/Cubic_spline/Subsystem1/Subsystem ==
  A : Inport
  B : Inport  Port=2
  c : Inport  Port=3
  f_x : Inport  Port=4
  Cubic_spline : Subsystem
  MatrixConcatenate : Concatenate  Mode=Multidimensional array  ConcatenateDimension=2
  Reshape : Reshape  OutputDimensionality=Column vector (2-D)
  Reshape1 : Reshape  OutputDimensionality=Column vector (2-D)
  j : Constant  Value=[0:0.09:10]
  1 : Outport
  wires:
  Reshape/1 -> MatrixConcatenate/1  "base_evaluation_1008_24b_Cubic_spline_Subsystem1_Subsystem_Reshape_1"
  j/1 -> Cubic_spline/1(j), Reshape/1  "base_evaluation_1008_24b_Cubic_spline_Subsystem1_Subsystem_j_1"
  Reshape1/1 -> MatrixConcatenate/2  "base_evaluation_1008_24b_Cubic_spline_Subsystem1_Subsystem_Reshape1_1"
  MatrixConcatenate/1 -> 1/1  "base_evaluation_1008_24b_Cubic_spline_Subsystem1_Subsystem_MatrixConcatenate_1"
  A/1 -> Cubic_spline/2(A)
  B/1 -> Cubic_spline/3(B)
  c/1 -> Cubic_spline/4(c)
  f_x/1 -> Cubic_spline/5(f_x)
  Cubic_spline/1(out) -> Reshape1/1

== system base_evaluation_1008_24b/Cubic_spline/Subsystem1/Subsystem1 ==
  A : Inport
  B : Inport  Port=2
  c : Inport  Port=3
  f_x : Inport  Port=4
  Cubic_spline : Subsystem
  MatrixConcatenate : Concatenate  Mode=Multidimensional array  ConcatenateDimension=2
  Reshape : Reshape  OutputDimensionality=Column vector (2-D)
  Reshape1 : Reshape  OutputDimensionality=Column vector (2-D)
  j : Constant  Value=[10:0.09:20.5]
  2 : Outport
  wires:
  Reshape/1 -> MatrixConcatenate/1  "base_evaluation_1008_24b_Cubic_spline_Subsystem1_Subsystem1_Reshape_1"
  j/1 -> Cubic_spline/1(j), Reshape/1  "base_evaluation_1008_24b_Cubic_spline_Subsystem1_Subsystem1_j_1"
  Reshape1/1 -> MatrixConcatenate/2  "base_evaluation_1008_24b_Cubic_spline_Subsystem1_Subsystem1_Reshape1_1"
  MatrixConcatenate/1 -> 2/1  "base_evaluation_1008_24b_Cubic_spline_Subsystem1_Subsystem1_MatrixConcatenate_1"
  A/1 -> Cubic_spline/2(A)
  B/1 -> Cubic_spline/3(B)
  c/1 -> Cubic_spline/4(c)
  f_x/1 -> Cubic_spline/5(f_x)
  Cubic_spline/1(out) -> Reshape1/1

== system base_evaluation_1008_24b/Cubic_spline/Subsystem1/Subsystem2 ==
  A : Inport
  B : Inport  Port=2
  c : Inport  Port=3
  f_x : Inport  Port=4
  Cubic_spline : Subsystem
  MatrixConcatenate : Concatenate  Mode=Multidimensional array  ConcatenateDimension=2
  Reshape : Reshape  OutputDimensionality=Column vector (2-D)
  Reshape1 : Reshape  OutputDimensionality=Column vector (2-D)
  j : Constant  Value=[20.5:0.09:35]
  3 : Outport
  wires:
  Reshape/1 -> MatrixConcatenate/1  "base_evaluation_1008_24b_Cubic_spline_Subsystem1_Subsystem2_Reshape_1"
  j/1 -> Cubic_spline/1(j), Reshape/1  "base_evaluation_1008_24b_Cubic_spline_Subsystem1_Subsystem2_j_1"
  Reshape1/1 -> MatrixConcatenate/2  "base_evaluation_1008_24b_Cubic_spline_Subsystem1_Subsystem2_Reshape1_1"
  MatrixConcatenate/1 -> 3/1  "base_evaluation_1008_24b_Cubic_spline_Subsystem1_Subsystem2_MatrixConcatenate_1"
  A/1 -> Cubic_spline/2(A)
  B/1 -> Cubic_spline/3(B)
  c/1 -> Cubic_spline/4(c)
  f_x/1 -> Cubic_spline/5(f_x)
  Cubic_spline/1(out) -> Reshape1/1

== system base_evaluation_1008_24b/Cubic_spline/Subsystem1/Subsystem3 ==
  A : Inport
  B : Inport  Port=2
  c : Inport  Port=3
  f_x : Inport  Port=4
  Cubic_spline : Subsystem
  MatrixConcatenate : Concatenate  Mode=Multidimensional array  ConcatenateDimension=2
  Reshape : Reshape  OutputDimensionality=Column vector (2-D)
  Reshape1 : Reshape  OutputDimensionality=Column vector (2-D)
  j : Constant  Value=[35:0.09:70.5]
  4 : Outport
  wires:
  Reshape/1 -> MatrixConcatenate/1  "base_evaluation_1008_24b_Cubic_spline_Subsystem1_Subsystem3_Reshape_1"
  j/1 -> Cubic_spline/1(j), Reshape/1  "base_evaluation_1008_24b_Cubic_spline_Subsystem1_Subsystem3_j_1"
  Reshape1/1 -> MatrixConcatenate/2  "base_evaluation_1008_24b_Cubic_spline_Subsystem1_Subsystem3_Reshape1_1"
  MatrixConcatenate/1 -> 4/1  "base_evaluation_1008_24b_Cubic_spline_Subsystem1_Subsystem3_MatrixConcatenate_1"
  A/1 -> Cubic_spline/2(A)
  B/1 -> Cubic_spline/3(B)
  c/1 -> Cubic_spline/4(c)
  f_x/1 -> Cubic_spline/5(f_x)
  Cubic_spline/1(out) -> Reshape1/1

== system base_evaluation_1008_24b/Cubic_spline/Subsystem1/Subsystem4 ==
  A : Inport
  B : Inport  Port=2
  c : Inport  Port=3
  f_x : Inport  Port=4
  Cubic_spline : Subsystem
  MatrixConcatenate : Concatenate  Mode=Multidimensional array  ConcatenateDimension=2
  Reshape : Reshape  OutputDimensionality=Column vector (2-D)
  Reshape1 : Reshape  OutputDimensionality=Column vector (2-D)
  j : Constant  Value=[70.5:0.09:100]
  5 : Outport
  wires:
  Reshape/1 -> MatrixConcatenate/1  "base_evaluation_1008_24b_Cubic_spline_Subsystem1_Subsystem4_Reshape_1"
  j/1 -> Cubic_spline/1(j), Reshape/1  "base_evaluation_1008_24b_Cubic_spline_Subsystem1_Subsystem4_j_1"
  Reshape1/1 -> MatrixConcatenate/2  "base_evaluation_1008_24b_Cubic_spline_Subsystem1_Subsystem4_Reshape1_1"
  MatrixConcatenate/1 -> 5/1  "base_evaluation_1008_24b_Cubic_spline_Subsystem1_Subsystem4_MatrixConcatenate_1"
  A/1 -> Cubic_spline/2(A)
  B/1 -> Cubic_spline/3(B)
  c/1 -> Cubic_spline/4(c)
  f_x/1 -> Cubic_spline/5(f_x)
  Cubic_spline/1(out) -> Reshape1/1

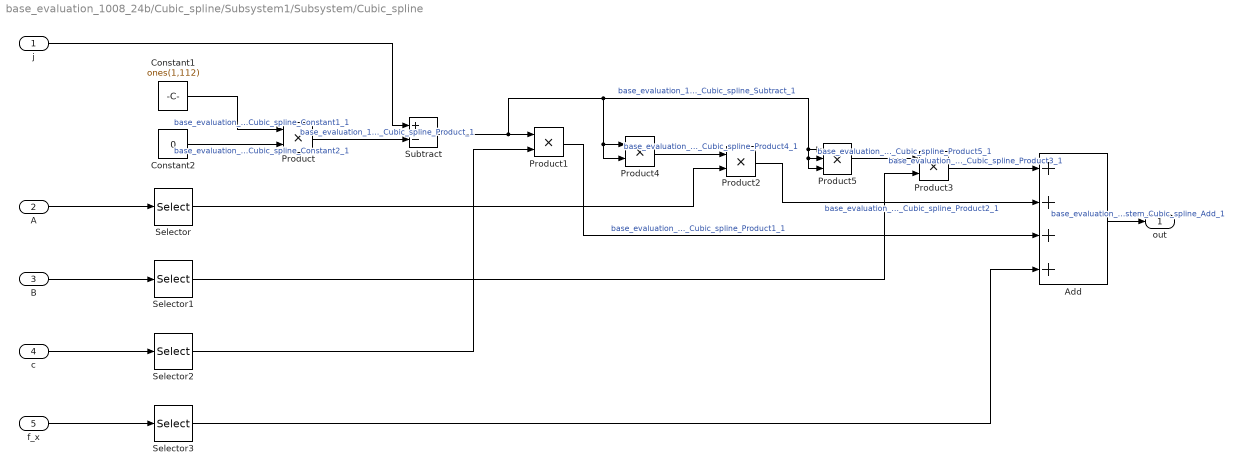
== system base_evaluation_1008_24b/Cubic_spline/Subsystem1/Subsystem/Cubic_spline ==
  j : Inport
  A : Inport  Port=2
  B : Inport  Port=3
  c : Inport  Port=4
  f_x : Inport  Port=5
  Add : Sum  Inputs=++++
  Constant1 : Constant  Value=ones(1,112)
  Constant2 : Constant  Value=0
  Product{,1..4} (5 alike) : Product
  Product5 : Product  Inputs=3
  Selector : Selector  InputPortWidth=5  IndexOptions=Index vector (dialog)  Indices=[1]  OutputSizes=1
  Selector1 : Selector  InputPortWidth=5  IndexOptions=Index vector (dialog)  Indices=[1]  OutputSizes=1
  Selector2 : Selector  InputPortWidth=5  IndexOptions=Index vector (dialog)  Indices=[1]  OutputSizes=1
  Selector3 : Selector  InputPortWidth=6  IndexOptions=Index vector (dialog)  Indices=[1]  OutputSizes=1
  Subtract : Sum  Inputs=+-
  out : Outport
  wires:
  c/1 -> Selector2/1
  Subtract/1 -> Product5/3, Product5/2, Product5/1, Product4/2, Product4/1, Product1/1  "base_evaluation_1008_24b_Cubic_spline_Subsystem1_Subsystem_Cubic_spline_Subtract_1"
  Product2/1 -> Add/2  "base_evaluation_1008_24b_Cubic_spline_Subsystem1_Subsystem_Cubic_spline_Product2_1"
  Constant2/1 -> Product/2  "base_evaluation_1008_24b_Cubic_spline_Subsystem1_Subsystem_Cubic_spline_Constant2_1"
  Product4/1 -> Product2/1  "base_evaluation_1008_24b_Cubic_spline_Subsystem1_Subsystem_Cubic_spline_Product4_1"
  Selector3/1 -> Add/4
  Product3/1 -> Add/1  "base_evaluation_1008_24b_Cubic_spline_Subsystem1_Subsystem_Cubic_spline_Product3_1"
  Selector1/1 -> Product3/2
  Constant1/1 -> Product/1  "base_evaluation_1008_24b_Cubic_spline_Subsystem1_Subsystem_Cubic_spline_Constant1_1"
  Selector2/1 -> Product1/2
  Product5/1 -> Product3/1  "base_evaluation_1008_24b_Cubic_spline_Subsystem1_Subsystem_Cubic_spline_Product5_1"
  Product1/1 -> Add/3  "base_evaluation_1008_24b_Cubic_spline_Subsystem1_Subsystem_Cubic_spline_Product1_1"
  Selector/1 -> Product2/2
  Product/1 -> Subtract/2  "base_evaluation_1008_24b_Cubic_spline_Subsystem1_Subsystem_Cubic_spline_Product_1"
  j/1 -> Subtract/1
  Add/1 -> out/1  "base_evaluation_1008_24b_Cubic_spline_Subsystem1_Subsystem_Cubic_spline_Add_1"
  A/1 -> Selector/1
  f_x/1 -> Selector3/1
  B/1 -> Selector1/1

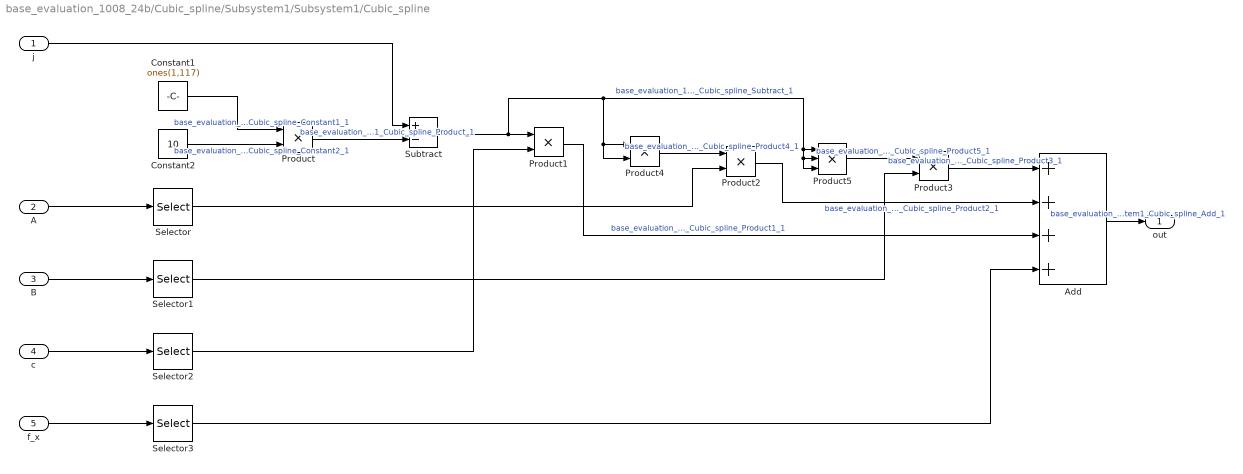
== system base_evaluation_1008_24b/Cubic_spline/Subsystem1/Subsystem1/Cubic_spline ==
  j : Inport
  A : Inport  Port=2
  B : Inport  Port=3
  c : Inport  Port=4
  f_x : Inport  Port=5
  Add : Sum  Inputs=++++
  Constant1 : Constant  Value=ones(1,117)
  Constant2 : Constant  Value=10
  Product{,1..4} (5 alike) : Product
  Product5 : Product  Inputs=3
  Selector : Selector  InputPortWidth=5  IndexOptions=Index vector (dialog)  Indices=[2]  OutputSizes=1
  Selector1 : Selector  InputPortWidth=5  IndexOptions=Index vector (dialog)  Indices=[2]  OutputSizes=1
  Selector2 : Selector  InputPortWidth=5  IndexOptions=Index vector (dialog)  Indices=[2]  OutputSizes=1
  Selector3 : Selector  InputPortWidth=6  IndexOptions=Index vector (dialog)  Indices=[2]  OutputSizes=1
  Subtract : Sum  Inputs=+-
  out : Outport
  wires:
  c/1 -> Selector2/1
  Subtract/1 -> Product5/3, Product5/2, Product5/1, Product4/2, Product4/1, Product1/1  "base_evaluation_1008_24b_Cubic_spline_Subsystem1_Subsystem1_Cubic_spline_Subtract_1"
  Product2/1 -> Add/2  "base_evaluation_1008_24b_Cubic_spline_Subsystem1_Subsystem1_Cubic_spline_Product2_1"
  Constant2/1 -> Product/2  "base_evaluation_1008_24b_Cubic_spline_Subsystem1_Subsystem1_Cubic_spline_Constant2_1"
  Product4/1 -> Product2/1  "base_evaluation_1008_24b_Cubic_spline_Subsystem1_Subsystem1_Cubic_spline_Product4_1"
  Selector3/1 -> Add/4
  Product3/1 -> Add/1  "base_evaluation_1008_24b_Cubic_spline_Subsystem1_Subsystem1_Cubic_spline_Product3_1"
  Selector1/1 -> Product3/2
  Constant1/1 -> Product/1  "base_evaluation_1008_24b_Cubic_spline_Subsystem1_Subsystem1_Cubic_spline_Constant1_1"
  Selector2/1 -> Product1/2
  Product5/1 -> Product3/1  "base_evaluation_1008_24b_Cubic_spline_Subsystem1_Subsystem1_Cubic_spline_Product5_1"
  Product1/1 -> Add/3  "base_evaluation_1008_24b_Cubic_spline_Subsystem1_Subsystem1_Cubic_spline_Product1_1"
  Selector/1 -> Product2/2
  Product/1 -> Subtract/2  "base_evaluation_1008_24b_Cubic_spline_Subsystem1_Subsystem1_Cubic_spline_Product_1"
  j/1 -> Subtract/1
  Add/1 -> out/1  "base_evaluation_1008_24b_Cubic_spline_Subsystem1_Subsystem1_Cubic_spline_Add_1"
  A/1 -> Selector/1
  f_x/1 -> Selector3/1
  B/1 -> Selector1/1

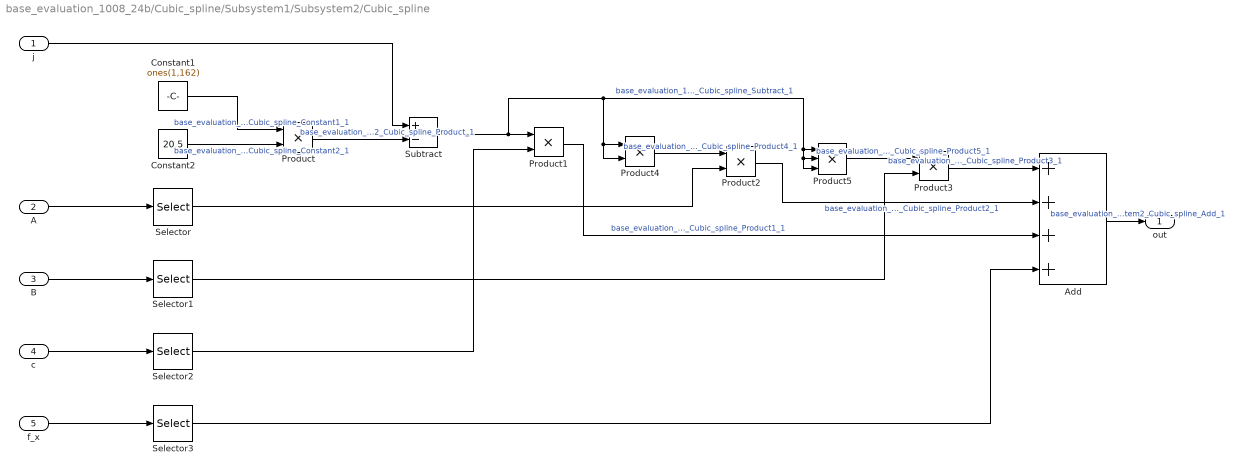
== system base_evaluation_1008_24b/Cubic_spline/Subsystem1/Subsystem2/Cubic_spline ==
  j : Inport
  A : Inport  Port=2
  B : Inport  Port=3
  c : Inport  Port=4
  f_x : Inport  Port=5
  Add : Sum  Inputs=++++
  Constant1 : Constant  Value=ones(1,162)
  Constant2 : Constant  Value=20.5
  Product{,1..4} (5 alike) : Product
  Product5 : Product  Inputs=3
  Selector : Selector  InputPortWidth=5  IndexOptions=Index vector (dialog)  Indices=[3]  OutputSizes=1
  Selector1 : Selector  InputPortWidth=5  IndexOptions=Index vector (dialog)  Indices=[3]  OutputSizes=1
  Selector2 : Selector  InputPortWidth=5  IndexOptions=Index vector (dialog)  Indices=[3]  OutputSizes=1
  Selector3 : Selector  InputPortWidth=6  IndexOptions=Index vector (dialog)  Indices=[3]  OutputSizes=1
  Subtract : Sum  Inputs=+-
  out : Outport
  wires:
  c/1 -> Selector2/1
  Subtract/1 -> Product5/3, Product5/2, Product5/1, Product4/1, Product4/2, Product1/1  "base_evaluation_1008_24b_Cubic_spline_Subsystem1_Subsystem2_Cubic_spline_Subtract_1"
  Product2/1 -> Add/2  "base_evaluation_1008_24b_Cubic_spline_Subsystem1_Subsystem2_Cubic_spline_Product2_1"
  Constant2/1 -> Product/2  "base_evaluation_1008_24b_Cubic_spline_Subsystem1_Subsystem2_Cubic_spline_Constant2_1"
  Product4/1 -> Product2/1  "base_evaluation_1008_24b_Cubic_spline_Subsystem1_Subsystem2_Cubic_spline_Product4_1"
  Selector3/1 -> Add/4
  Product3/1 -> Add/1  "base_evaluation_1008_24b_Cubic_spline_Subsystem1_Subsystem2_Cubic_spline_Product3_1"
  Selector1/1 -> Product3/2
  Constant1/1 -> Product/1  "base_evaluation_1008_24b_Cubic_spline_Subsystem1_Subsystem2_Cubic_spline_Constant1_1"
  Selector2/1 -> Product1/2
  Product5/1 -> Product3/1  "base_evaluation_1008_24b_Cubic_spline_Subsystem1_Subsystem2_Cubic_spline_Product5_1"
  Product1/1 -> Add/3  "base_evaluation_1008_24b_Cubic_spline_Subsystem1_Subsystem2_Cubic_spline_Product1_1"
  Selector/1 -> Product2/2
  Product/1 -> Subtract/2  "base_evaluation_1008_24b_Cubic_spline_Subsystem1_Subsystem2_Cubic_spline_Product_1"
  j/1 -> Subtract/1
  Add/1 -> out/1  "base_evaluation_1008_24b_Cubic_spline_Subsystem1_Subsystem2_Cubic_spline_Add_1"
  A/1 -> Selector/1
  f_x/1 -> Selector3/1
  B/1 -> Selector1/1

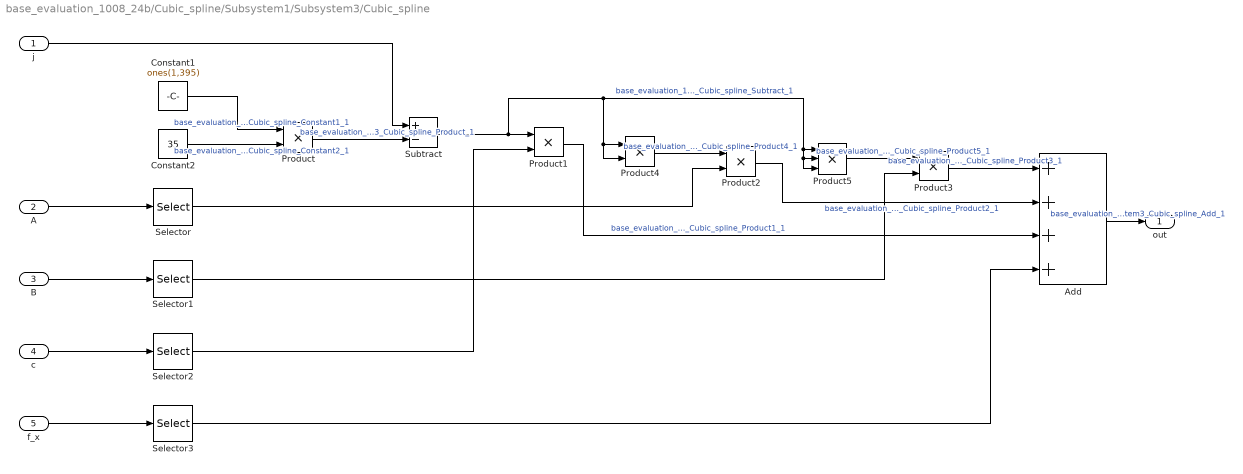
== system base_evaluation_1008_24b/Cubic_spline/Subsystem1/Subsystem3/Cubic_spline ==
  j : Inport
  A : Inport  Port=2
  B : Inport  Port=3
  c : Inport  Port=4
  f_x : Inport  Port=5
  Add : Sum  Inputs=++++
  Constant1 : Constant  Value=ones(1,395)
  Constant2 : Constant  Value=35
  Product{,1..4} (5 alike) : Product
  Product5 : Product  Inputs=3
  Selector : Selector  InputPortWidth=5  IndexOptions=Index vector (dialog)  Indices=[4]  OutputSizes=1
  Selector1 : Selector  InputPortWidth=5  IndexOptions=Index vector (dialog)  Indices=[4]  OutputSizes=1
  Selector2 : Selector  InputPortWidth=5  IndexOptions=Index vector (dialog)  Indices=[4]  OutputSizes=1
  Selector3 : Selector  InputPortWidth=6  IndexOptions=Index vector (dialog)  Indices=[4]  OutputSizes=1
  Subtract : Sum  Inputs=+-
  out : Outport
  wires:
  c/1 -> Selector2/1
  Subtract/1 -> Product5/3, Product5/2, Product5/1, Product4/2, Product4/1, Product1/1  "base_evaluation_1008_24b_Cubic_spline_Subsystem1_Subsystem3_Cubic_spline_Subtract_1"
  Product2/1 -> Add/2  "base_evaluation_1008_24b_Cubic_spline_Subsystem1_Subsystem3_Cubic_spline_Product2_1"
  Constant2/1 -> Product/2  "base_evaluation_1008_24b_Cubic_spline_Subsystem1_Subsystem3_Cubic_spline_Constant2_1"
  Product4/1 -> Product2/1  "base_evaluation_1008_24b_Cubic_spline_Subsystem1_Subsystem3_Cubic_spline_Product4_1"
  Selector3/1 -> Add/4
  Product3/1 -> Add/1  "base_evaluation_1008_24b_Cubic_spline_Subsystem1_Subsystem3_Cubic_spline_Product3_1"
  Selector1/1 -> Product3/2
  Constant1/1 -> Product/1  "base_evaluation_1008_24b_Cubic_spline_Subsystem1_Subsystem3_Cubic_spline_Constant1_1"
  Selector2/1 -> Product1/2
  Product5/1 -> Product3/1  "base_evaluation_1008_24b_Cubic_spline_Subsystem1_Subsystem3_Cubic_spline_Product5_1"
  Product1/1 -> Add/3  "base_evaluation_1008_24b_Cubic_spline_Subsystem1_Subsystem3_Cubic_spline_Product1_1"
  Selector/1 -> Product2/2
  Product/1 -> Subtract/2  "base_evaluation_1008_24b_Cubic_spline_Subsystem1_Subsystem3_Cubic_spline_Product_1"
  j/1 -> Subtract/1
  Add/1 -> out/1  "base_evaluation_1008_24b_Cubic_spline_Subsystem1_Subsystem3_Cubic_spline_Add_1"
  A/1 -> Selector/1
  f_x/1 -> Selector3/1
  B/1 -> Selector1/1

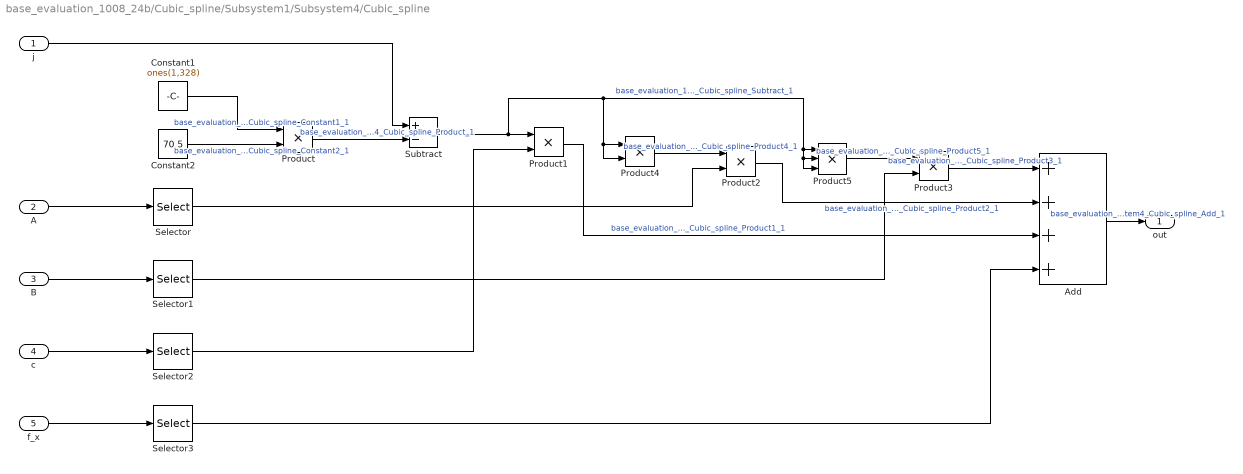
== system base_evaluation_1008_24b/Cubic_spline/Subsystem1/Subsystem4/Cubic_spline ==
  j : Inport
  A : Inport  Port=2
  B : Inport  Port=3
  c : Inport  Port=4
  f_x : Inport  Port=5
  Add : Sum  Inputs=++++
  Constant1 : Constant  Value=ones(1,328)
  Constant2 : Constant  Value=70.5
  Product{,1..4} (5 alike) : Product
  Product5 : Product  Inputs=3
  Selector : Selector  InputPortWidth=5  IndexOptions=Index vector (dialog)  Indices=[5]  OutputSizes=1
  Selector1 : Selector  InputPortWidth=5  IndexOptions=Index vector (dialog)  Indices=[5]  OutputSizes=1
  Selector2 : Selector  InputPortWidth=5  IndexOptions=Index vector (dialog)  Indices=[5]  OutputSizes=1
  Selector3 : Selector  InputPortWidth=6  IndexOptions=Index vector (dialog)  Indices=[5]  OutputSizes=1
  Subtract : Sum  Inputs=+-
  out : Outport
  wires:
  c/1 -> Selector2/1
  Subtract/1 -> Product5/3, Product5/2, Product5/1, Product4/2, Product4/1, Product1/1  "base_evaluation_1008_24b_Cubic_spline_Subsystem1_Subsystem4_Cubic_spline_Subtract_1"
  Product2/1 -> Add/2  "base_evaluation_1008_24b_Cubic_spline_Subsystem1_Subsystem4_Cubic_spline_Product2_1"
  Constant2/1 -> Product/2  "base_evaluation_1008_24b_Cubic_spline_Subsystem1_Subsystem4_Cubic_spline_Constant2_1"
  Product4/1 -> Product2/1  "base_evaluation_1008_24b_Cubic_spline_Subsystem1_Subsystem4_Cubic_spline_Product4_1"
  Selector3/1 -> Add/4
  Product3/1 -> Add/1  "base_evaluation_1008_24b_Cubic_spline_Subsystem1_Subsystem4_Cubic_spline_Product3_1"
  Selector1/1 -> Product3/2
  Constant1/1 -> Product/1  "base_evaluation_1008_24b_Cubic_spline_Subsystem1_Subsystem4_Cubic_spline_Constant1_1"
  Selector2/1 -> Product1/2
  Product5/1 -> Product3/1  "base_evaluation_1008_24b_Cubic_spline_Subsystem1_Subsystem4_Cubic_spline_Product5_1"
  Product1/1 -> Add/3  "base_evaluation_1008_24b_Cubic_spline_Subsystem1_Subsystem4_Cubic_spline_Product1_1"
  Selector/1 -> Product2/2
  Product/1 -> Subtract/2  "base_evaluation_1008_24b_Cubic_spline_Subsystem1_Subsystem4_Cubic_spline_Product_1"
  j/1 -> Subtract/1
  Add/1 -> out/1  "base_evaluation_1008_24b_Cubic_spline_Subsystem1_Subsystem4_Cubic_spline_Add_1"
  A/1 -> Selector/1
  f_x/1 -> Selector3/1
  B/1 -> Selector1/1
